simulink model "QAM64_class"  (R2019a)
settings: Solver=VariableStepAuto  StartTime=0.0  StopTime=10.0  RelTol=1e-3  EnableMultiTasking=on
values from neighbouring files (symbols this model uses):
  M_64 = 64    [Performance.m]
  Tsym_64 = (1/Rb) *log2(M_64)    [Performance.m]
libraries: commdigbbndam3 x2, commchan3 x1, commsink2 x1, commutil2 x1, commrandsrc3 x1
settings Model: Creator=hussein  LastModifiedBy=Administrator
settings DataIOCC: ReturnWorkspaceOutputs=off
settings OptimizationCC: LifeSpan=inf
settings DebuggingCC: SFUnexpectedBacktrackingDiag=warning  SFNoUnconditionalDefaultTransitionDiag=warning  ArithmeticOperatorsInVariantConditions=warning
settings SFSimCC: SimUseLocalCustomCode=off
settings RTWCC: RTWUseLocalCustomCode=off
settings CodeAppCC: StateflowObjectComments=on
settings GRTTargetCC: TargetLangStandard=C89/C90 (ANSI)  GeneratePreprocessorConditionals=Disable all
settings ConfigComp: CovMetricSettings=dw  CovHtmlReporting=on  CovSaveCumulativeToWorkspaceVar=on  CovSaveSingleToWorkspaceVar=on  CovExternalEMLEnable=off

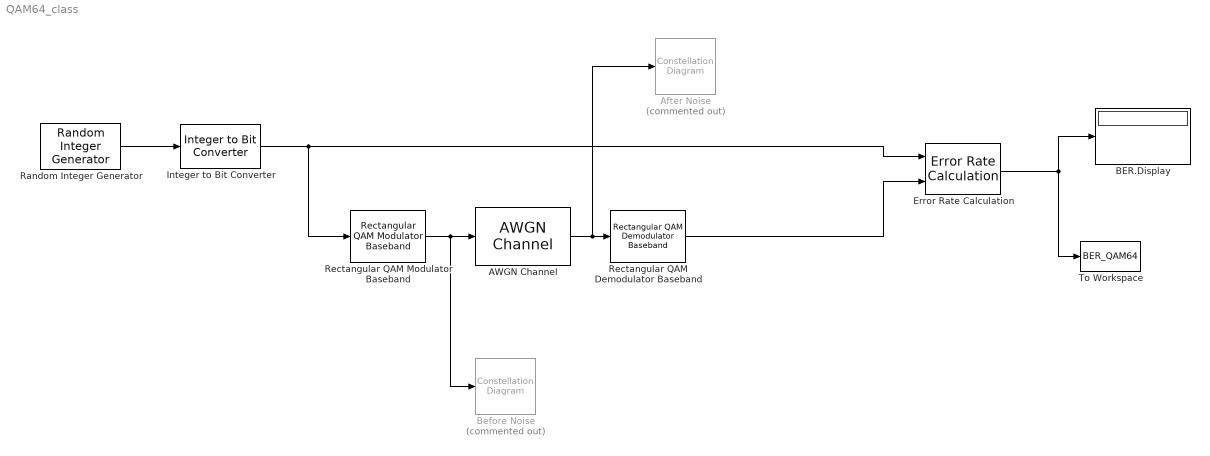
== system QAM64_class ==
  AWGN Channel : commchan3/AWGN Channel  InputProcessing=Columns as channels (frame based)  seed=67  noiseMode="Signal to noise ratio  (Eb/No)"  EbNodB=EbNo  EsNodB=10  SNRdB=10  bitsPerSym=log2(M_64)  Ps=1  Tsym=Tsym_64  variance=1
      settings: SourceProductName=Communications Toolbox
  After Noise : ConstellationDiagram  Commented=on
  "BER.Display " : Display
  Before Noise : ConstellationDiagram  Commented=on
  Error Rate Calculation : commsink2/Error Rate Calculation  N=0  st_delay=0  cp_mode=Entire frame  subframe=[]  PMode=Port  WsName=ErrorVec  RsMode2=off  stop=on  numErr=maxNumErrs  maxBits=maxNumBits
      settings: SourceProductName=Communications Toolbox
  Integer to Bit Converter : commutil2/Integer to Bit Converter  nbits=log2(M_64)  signedInputValues=Unsigned  bitOrder=MSB first  outDtype=Smallest unsigned integer
      settings: SourceProductName=Communications Toolbox
  Random Integer Generator : commrandsrc3/Random Integer Generator  SetSize=M_64  SeedSource=Parameter  Seed=529558  SampleTime=Tsym_64  SamplesPerFrame=100  OutputDataType=uint8  SimulateUsing=Interpreted execution
      settings: SourceProductName=Communications Toolbox
  Rectangular QAM Demodulator Baseband : commdigbbndam3/Rectangular QAM Demodulator Baseband  M=M_64  OutType=Bit  DecType=Hard decision  VarSource=Dialog  Variance=1  Dec=Gray  Mapping=[0:15]  PowType=Average Power  MinDist=2  AvgPow=1  PeakPow=1  Ph=0  outDtype1=Inherit via internal rule  outDtype2=Inherit via internal rule  derotateFactorWordLen=16  derotateFactorDataTypeStr=Inherit: Same word length as input  derotateFactorLastDataTypeStr=Inherit: Same word length as input  denormFactorWordLen=16  denormFactorDataTypeStr=Inherit: Same word length as input  denormFactorLastDataTypeStr=Inherit: Same word length as input  prodOutWordLen=32  prodOutOverflowMode=Wrap  prodOutRoundingMode=Floor  prodOutOvFlMode=off  prodOutOvFlModeLastStrValue=off  sumWordLen=32
      settings: SourceProductName=Communications Toolbox
  Rectangular QAM Modulator Baseband : commdigbbndam3/Rectangular QAM Modulator Baseband  M=M_64  InType=Bit  Enc=Gray  Mapping=[0:15]  PowType=Average Power  MinDist=2  AvgPow=1  PeakPow=1  Ph=0  outDtype=double  outWordLen=16  outUDDataType=sfix(16)  outFracLenMode=Best precision  outFracLen=15  outDataTypeStr=double  outLastDataTypeStr=double
      settings: SourceProductName=Communications Toolbox
  To Workspace : ToWorkspace  VariableName=BER_QAM64  SampleTime=-1
      settings: MaxDataPoints=1  Save2DSignal=2-D array (concatenate along first dimension)
  wires:
  Random Integer Generator/1 -> Integer to Bit Converter/1
  Rectangular QAM Modulator Baseband/1 -> Before Noise/1, AWGN Channel/1
  AWGN Channel/1 -> Rectangular QAM Demodulator Baseband/1, After Noise/1
  Rectangular QAM Demodulator Baseband/1 -> Error Rate Calculation/2
  Error Rate Calculation/1 -> "BER.Display "/1, To Workspace/1
  Integer to Bit Converter/1 -> Error Rate Calculation/1, Rectangular QAM Modulator Baseband/1
